simulink model "PlaneSimulationModel_withSensors_r17"  (R2022b)
settings: Solver=FixedStepAuto  StartTime=0.0  StopTime=20  FixedStep=0.0025  RelTol=1e-3
libraries: simulink x12
(part 1 of 2)
settings Model: DataDictionary=plane_sm_dictionary.sldd  EnableAccessToBaseWorkspace=off  PauseTimes=0  Creator=Marcin  LastModifiedBy=Wojtek
settings SolverCC: AlgebraicLoopSolver=TrustRegion
settings DataIOCC: ReturnWorkspaceOutputs=off
settings OptimizationCC: DefaultParameterBehavior=Inlined  UseDivisionForNetSlopeComputation=on  DefaultUnderspecifiedDataType=single  PassReuseOutputArgsAs=Individual arguments  EfficientTunableParamExpr=on
settings DebuggingCC: ParameterPrecisionLossMsg=none  ParameterTunabilityLossMsg=error  UnconnectedInputMsg=warning  UnconnectedOutputMsg=warning  UnconnectedLineMsg=warning  SFMachineParentedDataDiag=warning  ArithmeticOperatorsInVariantConditions=warning
settings HardwareCC: ProdBitPerPointer=32  ProdBitPerSizeT=32  ProdBitPerPtrDiffT=32  ProdLargestAtomicInteger=Long  ProdLargestAtomicFloat=Double  ProdWordSize=32  ProdHWDeviceType=ARM Compatible->ARM Cortex-M
settings ModelReferenceCC: EnableRefExpFcnMdlSchedulingChecks=on
settings SFSimCC: SimUseLocalCustomCode=off  MATLABDynamicMemAlloc=off  CustomCodeUndefinedFunction=UseInterfaceOnly
settings RTWCC: Description=Embedded Coder  SystemTargetFile=ert.tlc  TemplateMakefile=ert_default_tmf  GenerateReport=on  RTWUseLocalCustomCode=off  Toolchain=MinGW64 | gmake (64-bit Windows)  IncludeHyperlinkInReport=on  LaunchReport=on  GenerateTraceInfo=on  GenerateTraceReport=on  GenerateTraceReportSl=on  GenerateTraceReportSf=on  GenerateTraceReportEml=on
settings CodeAppCC: ForceParamTrailComments=on  OperatorAnnotations=on  SimulinkDataObjDesc=on  SFDataObjDesc=on  InsertBlockDesc=on
settings ERTTargetCC: TargetLangStandard=C99 (ISO)  CodeReplacementLibrary=GNU C99 extensions  SupportVariableSizeSignals=on  InlinedParameterPlacement=NonHierarchical  ERTCustomFileTemplate=example_file_process.tlc  MemSecPackage=Simulink

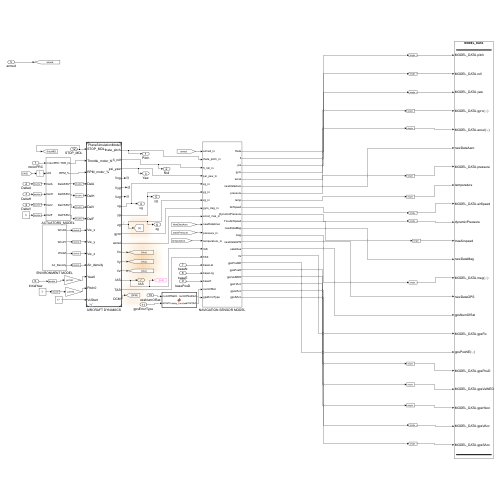
[thumbnail: Simulink's stored preview of the top-level diagram]
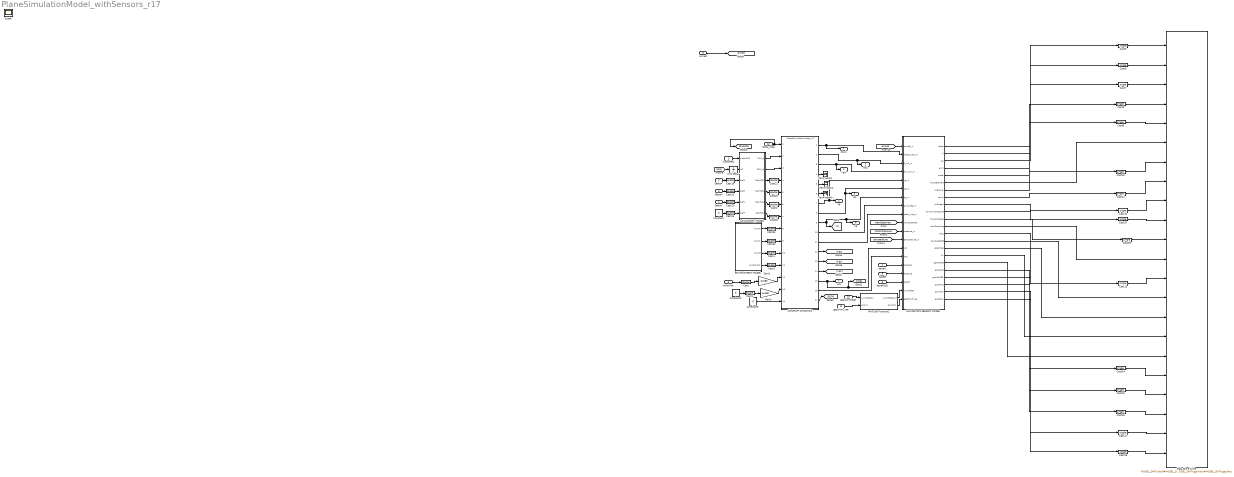
== system PlaneSimulationModel_withSensors_r17 ==
  motorPRC : Inport
  DeltaA : Inport  Port=2
  DeltaH : Inport  Port=3
  DeltaV : Inport  Port=4
  armed : Inport  Port=5  OutDataTypeStr=boolean
  InitialYaw : Inport  Port=6
  baseN : Inport  Port=7
  baseE : Inport  Port=8
  basePosD : Inport  Port=9
  gpsNumOfSat : Inport  Port=10  OutDataTypeStr=uint8
  gpsErrorType : Inport  Port=11  OutDataTypeStr=uint8
  STOP_MDL : Inport  Port=12
  ACTUATORS_MODEL : Subsystem
  AIRCRAFT DYNAMICS : ModelReference  Priority=10  ModelNameDialog=PlaneSimulationModel_r17.slx  SimulationMode=Normal  ModelReferenceVersion=11.9
  Cast{,1..4,19..24,30..32} (14 alike) : DataTypeConversion  OutDataTypeStr=double  SaturateOnIntegerOverflow=off  RndMeth=Floor
  Cast{5..18,33,37} (16 alike) : DataTypeConversion  OutDataTypeStr=single  SaturateOnIntegerOverflow=off  RndMeth=Floor
  Constant : Constant  Value=0
  Constant2 : Constant  Value=3  OutDataTypeStr=single  SampleTime=-1
  Constant6 : Constant  Value=17  OutDataTypeStr=double  SampleTime=-1
  Data Store Write : DataStoreWrite  DataStoreName=MODEL_DATA  DataStoreElements=MODEL_DATA.pitch#MODEL_DATA.roll#MODEL_DATA.yaw#MODEL_DATA.gyro(:,:)#MODEL_DATA.accel(:,:)#MODEL_DATA.newDateAero#MODEL_DATA.pressure#MODEL_DATA.temperature#MODEL_DATA.airSpeed#MODEL_DATA.dynamicPressure#MODEL_DATA.trueAirspeed#MODEL_DATA.newDataMag#MODEL_DATA.mag(:,:)#MODEL_DATA.newDataGPS#MODEL_DATA.gpsNumOfSat#MODEL_DATA.gpsFix#MODEL_DATA.gpsPosNE(:,:)#MODEL_DATA.gpsPosD#MODEL_DATA.gpsVelNED#MODEL_DATA.gpsHAcc#MODEL_DATA.gpsVAcc#MODEL_DATA.gpsSAcc  IndexOptions=Index vector (dialog)  Indices=1  OutputSizes=1
  ENVIRONMENT MODEL : Subsystem
  Gain2 : Gain  Gain=pi/180
  Gain3 : Gain  Gain=pi/180
  MATLAB Function2 : MATLAB Function  TreatAsAtomicUnit=on
  NAVIGATION SENSOR MODEL : Subsystem  Priority=50
  Terminator1 : Terminator
  Terminator2 : Terminator
  Terminator3 : Terminator
  Unit Delay : UnitDelay  SampleTime=-1  HasFrameUpgradeWarning=on
  Pitch : Outport
  Roll : Outport  Port=2
  Yaw : Outport  Port=3
  xg : Outport  Port=4
  yg : Outport  Port=5
  zg : Outport  Port=6
  IAS : Outport  Port=7
  Scope : Scope
  tag scope: StopMDL=global, armed=global
  wires:
  AIRCRAFT DYNAMICS/14 -> [Vez]
  Cast12/1 -> Data Store Write/9
  AIRCRAFT DYNAMICS/16 -> NAVIGATION SENSOR MODEL/14(TAS)
  MATLAB Function2/2(errorOut) -> NAVIGATION SENSOR MODEL/19(gpsErrorType)
  NAVIGATION SENSOR MODEL/2(fi) -> Cast6/1
  NAVIGATION SENSOR MODEL/5(accel) -> Cast9/1
  MATLAB Function2/1(numOfSatOut) -> NAVIGATION SENSOR MODEL/18(numOfSat)
  STOP_MDL/1 -> [StopMDL], AIRCRAFT DYNAMICS/1
  Cast18/1 -> Data Store Write/22
  Cast11/1 -> Data Store Write/8
  AIRCRAFT DYNAMICS/15 -> IAS/1, NAVIGATION SENSOR MODEL/13(IAS), [IAS]
  Cast33/1 -> Data Store Write/11
  baseE/1 -> NAVIGATION SENSOR MODEL/16(baseLng)
  NAVIGATION SENSOR MODEL/17(gpsPosNE) -> Data Store Write/17
  Constant6/1 -> AIRCRAFT DYNAMICS/14
  NAVIGATION SENSOR MODEL/18(gpsPosD) -> Cast14/1
  AIRCRAFT DYNAMICS/17 -> [DCM]
  NAVIGATION SENSOR MODEL/13(mag) -> Cast13/1
  AIRCRAFT DYNAMICS/12 -> [Vex]
  Cast20/1 -> AIRCRAFT DYNAMICS/5
  Cast10/1 -> Data Store Write/7
  [IAS] -> Unit Delay/1
  AIRCRAFT DYNAMICS/1 -> NAVIGATION SENSOR MODEL/2(theta_pitch_in), Pitch/1
  AIRCRAFT DYNAMICS/2 -> Roll/1, NAVIGATION SENSOR MODEL/3(fi_roll_in)
  Cast/1 -> Gain2/1
  AIRCRAFT DYNAMICS/3 -> NAVIGATION SENSOR MODEL/4(psi_yaw_in), Yaw/1
  [armed] -> NAVIGATION SENSOR MODEL/1(armed_in)
  AIRCRAFT DYNAMICS/7 -> NAVIGATION SENSOR MODEL/5(xg_in), xg/1
  [staticPressure] -> NAVIGATION SENSOR MODEL/11(pressure_in)
  AIRCRAFT DYNAMICS/11 -> NAVIGATION SENSOR MODEL/9(accel_mss_in)
  AIRCRAFT DYNAMICS/10 -> NAVIGATION SENSOR MODEL/8(gyro_deg_in)
  AIRCRAFT DYNAMICS/9 -> [z], NAVIGATION SENSOR MODEL/7(zg_in), zg/1
  NAVIGATION SENSOR MODEL/21(gpsVAcc) -> Cast17/1
  AIRCRAFT DYNAMICS/8 -> NAVIGATION SENSOR MODEL/6(yg_in), yg/1
  NAVIGATION SENSOR MODEL/4(gyro) -> Cast8/1
  gpsNumOfSat/1 -> MATLAB Function2/1(numOfSatIn)
  Cast16/1 -> Data Store Write/20
  Cast15/1 -> Data Store Write/19
  Cast13/1 -> Data Store Write/13
  Gain3/1 -> AIRCRAFT DYNAMICS/13
  Cast9/1 -> Data Store Write/5
  Cast8/1 -> Data Store Write/4
  Cast7/1 -> Data Store Write/3
  NAVIGATION SENSOR MODEL/11(TrueAirSpeed) -> Cast33/1
  NAVIGATION SENSOR MODEL/10(DynamicPressure) -> Cast37/1
  InitialYaw/1 -> Cast/1
  Cast5/1 -> Data Store Write/1
  NAVIGATION SENSOR MODEL/15(satellites) -> Data Store Write/15
  NAVIGATION SENSOR MODEL/20(gpsHAcc) -> Cast16/1
  NAVIGATION SENSOR MODEL/19(gpsVelNED) -> Cast15/1
  Cast1/1 -> Gain3/1
  NAVIGATION SENSOR MODEL/9(AirSpeed) -> Cast12/1
  NAVIGATION SENSOR MODEL/8(temp) -> Cast11/1
  NAVIGATION SENSOR MODEL/3(psi) -> Cast7/1
  NAVIGATION SENSOR MODEL/16(fix) -> Data Store Write/16
  [NewDataAreo] -> NAVIGATION SENSOR MODEL/10(newDataAreo)
  NAVIGATION SENSOR MODEL/7(pressure) -> Cast10/1
  NAVIGATION SENSOR MODEL/1(theta) -> Cast5/1
  NAVIGATION SENSOR MODEL/6(newDataAero) -> Data Store Write/6
  [temperature] -> NAVIGATION SENSOR MODEL/12(temperature_in)
  basePosD/1 -> NAVIGATION SENSOR MODEL/17(baseH)
  Cast14/1 -> Data Store Write/18
  Cast21/1 -> AIRCRAFT DYNAMICS/4
  Cast37/1 -> Data Store Write/10
  NAVIGATION SENSOR MODEL/12(newDataMag) -> Data Store Write/12
  NAVIGATION SENSOR MODEL/14(newDataGPS) -> Data Store Write/14
  gpsErrorType/1 -> MATLAB Function2/2(errorIn)
  Cast6/1 -> Data Store Write/2
  Constant2/1 -> Cast1/1
  AIRCRAFT DYNAMICS/13 -> [Vey]
  Cast17/1 -> Data Store Write/21
  baseN/1 -> NAVIGATION SENSOR MODEL/15(baseLat)
  NAVIGATION SENSOR MODEL/22(gpsSAcc) -> Cast18/1
  armed/1 -> [armed]
  AIRCRAFT DYNAMICS/4 -> Terminator1/1
  AIRCRAFT DYNAMICS/5 -> Terminator2/1
  AIRCRAFT DYNAMICS/6 -> Terminator3/1
  Cast2/1 -> AIRCRAFT DYNAMICS/6
  Gain2/1 -> AIRCRAFT DYNAMICS/12
  Cast4/1 -> AIRCRAFT DYNAMICS/10
  Cast32/1 -> AIRCRAFT DYNAMICS/9
  Cast31/1 -> AIRCRAFT DYNAMICS/8
  Cast30/1 -> AIRCRAFT DYNAMICS/7
  Cast3/1 -> AIRCRAFT DYNAMICS/11
  ENVIRONMENT MODEL/4(Air_Density) -> Cast3/1
  ENVIRONMENT MODEL/3(WindZ) -> Cast4/1
  ENVIRONMENT MODEL/2(WindY) -> Cast32/1
  ENVIRONMENT MODEL/1(WindX) -> Cast31/1
  motorPRC/1 -> ACTUATORS_MODEL/1(motorPRC)
  Unit Delay/1 -> ACTUATORS_MODEL/2(IAS)
  ACTUATORS_MODEL/1(THR_N) -> AIRCRAFT DYNAMICS/2
  ACTUATORS_MODEL/2(RPM_%) -> AIRCRAFT DYNAMICS/3
  ACTUATORS_MODEL/3(DelASRV) -> Cast21/1
  ACTUATORS_MODEL/4(DelHSRV) -> Cast20/1
  ACTUATORS_MODEL/5(DelVSRV) -> Cast2/1
  ACTUATORS_MODEL/6(DelFSRV) -> Cast30/1
  DeltaA/1 -> Cast19/1
  DeltaH/1 -> Cast22/1
  DeltaV/1 -> Cast23/1
  Constant/1 -> Cast24/1
  Cast19/1 -> ACTUATORS_MODEL/3(DelA)
  Cast22/1 -> ACTUATORS_MODEL/4(DelH)
  Cast23/1 -> ACTUATORS_MODEL/5(DelV)
  Cast24/1 -> ACTUATORS_MODEL/6(DelF)

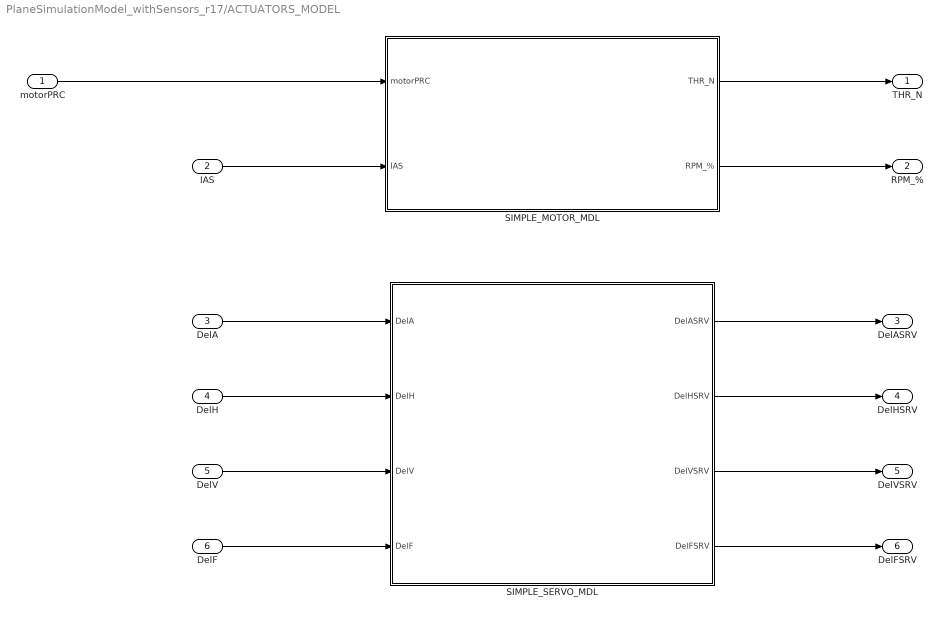
== system PlaneSimulationModel_withSensors_r17/ACTUATORS_MODEL ==
  motorPRC : Inport
  IAS : Inport  Port=2
  DelA : Inport  Port=3
  DelH : Inport  Port=4
  DelV : Inport  Port=5
  DelF : Inport  Port=6
  SIMPLE_MOTOR_MDL : Subsystem
  SIMPLE_SERVO_MDL : Subsystem
  THR_N : Outport
  RPM_% : Outport  Port=2
  DelASRV : Outport  Port=3
  DelHSRV : Outport  Port=4
  DelVSRV : Outport  Port=5
  DelFSRV : Outport  Port=6
  wires:
  SIMPLE_MOTOR_MDL/1(THR_N) -> THR_N/1
  SIMPLE_MOTOR_MDL/2(RPM_%) -> RPM_%/1
  IAS/1 -> SIMPLE_MOTOR_MDL/2(IAS)
  motorPRC/1 -> SIMPLE_MOTOR_MDL/1(motorPRC)
  DelA/1 -> SIMPLE_SERVO_MDL/1(DelA)
  SIMPLE_SERVO_MDL/1(DelASRV) -> DelASRV/1
  DelH/1 -> SIMPLE_SERVO_MDL/2(DelH)
  DelV/1 -> SIMPLE_SERVO_MDL/3(DelV)
  DelF/1 -> SIMPLE_SERVO_MDL/4(DelF)
  SIMPLE_SERVO_MDL/2(DelHSRV) -> DelHSRV/1
  SIMPLE_SERVO_MDL/3(DelVSRV) -> DelVSRV/1
  SIMPLE_SERVO_MDL/4(DelFSRV) -> DelFSRV/1

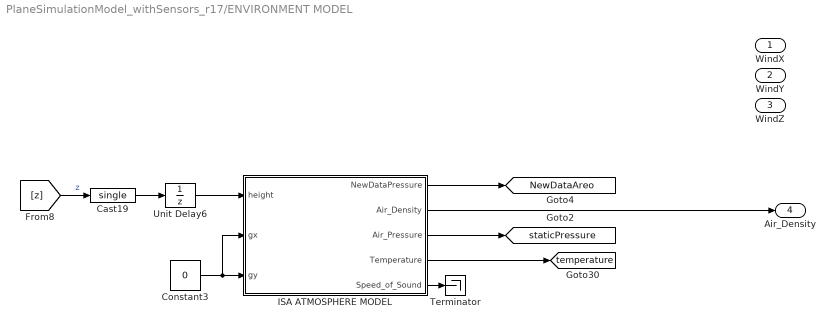
== system PlaneSimulationModel_withSensors_r17/ENVIRONMENT MODEL ==
  Cast19 : DataTypeConversion  OutDataTypeStr=single  SaturateOnIntegerOverflow=off  RndMeth=Floor
  Constant3 : Constant  Value=0  OutDataTypeStr=single  SampleTime=-1
  ISA ATMOSPHERE MODEL : MATLAB Function  TreatAsAtomicUnit=on  mask{acc_to_gravity=9.80665, ratio_heats=1.4, gas_const=287.0531, lapse_rate=0.0065, height_of_troposphere=110000, height_of_tropopause=20000, air_density=1.225, pressure_sea_level=101325, temperature_sea_level=288.15, lowest_altitude=0, frequency=100, delay=50, pressure_deviation=6, en_acc_pressure_noise=on, max_bias_value=0, max_bias_time=50, dt=0.0025}
      mask prompts: acc_to_gravity "Acceleration due to gravity (m/s^2)"; ratio_heats "Ratio of specific heats"; gas_const "Characteristic gas constant (J/Kg/K)"; lapse_rate "Lapse rate (K/m)"; height_of_troposphere "Height of troposphere (m)"; height_of_tropopause "Height of tropopause (m)"; air_density "Air density at mean sea level (Kg/m^3)"; pressure_sea_level "Ambient pressure at mean sea level (N/m^2)"; temperature_sea_level "Ambient temperature at mean sea level"; lowest_altitude "Lowest altitude (m)"; frequency "Frequency [Hz]"; delay "Latency [ms]"; pressure_deviation "Pressure Deviation [Pa]"; en_acc_pressure_noise "Enable acc pressure noise"; max_bias_value "Max pressure bias value [Pa]"; max_bias_time "Max value bias time [s]"; dt "Sample Time [s]"
  Terminator : Terminator
  Unit Delay6 : UnitDelay  SampleTime=-1  HasFrameUpgradeWarning=on
  WindX : Outport
  WindY : Outport  Port=2
  WindZ : Outport  Port=3
  Air_Density : Outport  Port=4
  tag scope: NewDataAreo=global, staticPressure=global, temperature=global
  wires:
  [z] -> Cast19/1  "z"
  ISA ATMOSPHERE MODEL/3(Air_Pressure) -> [staticPressure]
  Constant3/1 -> ISA ATMOSPHERE MODEL/2(gx), ISA ATMOSPHERE MODEL/3(gy)
  Unit Delay6/1 -> ISA ATMOSPHERE MODEL/1(height)
  ISA ATMOSPHERE MODEL/5(Speed_of_Sound) -> Terminator/1
  ISA ATMOSPHERE MODEL/1(NewDataPressure) -> [NewDataAreo]
  Cast19/1 -> Unit Delay6/1
  ISA ATMOSPHERE MODEL/4(Temperature) -> [temperature]
  ISA ATMOSPHERE MODEL/2(Air_Density) -> Air_Density/1

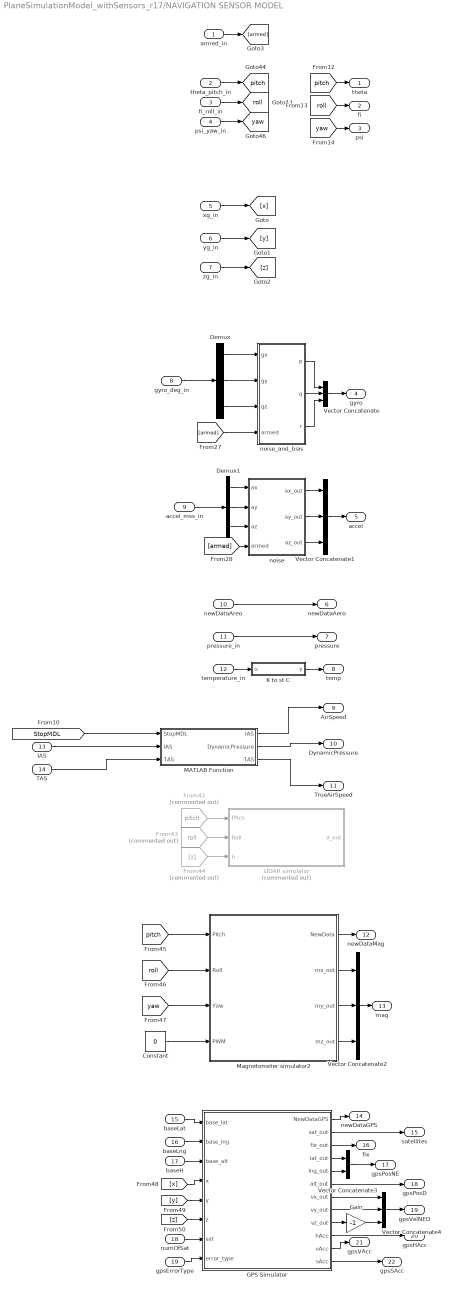
== system PlaneSimulationModel_withSensors_r17/NAVIGATION SENSOR MODEL ==
  armed_in : Inport
  theta_pitch_in : Inport  Port=2
  fi_roll_in : Inport  Port=3
  psi_yaw_in : Inport  Port=4
  xg_in : Inport  Port=5
  yg_in : Inport  Port=6
  zg_in : Inport  Port=7
  gyro_deg_in : Inport  Port=8
  accel_mss_in : Inport  Port=9
  newDataAreo : Inport  Port=10
  pressure_in : Inport  Port=11
  temperature_in : Inport  Port=12
  IAS : Inport  Port=13
  TAS : Inport  Port=14
  baseLat : Inport  Port=15
  baseLng : Inport  Port=16
  baseH : Inport  Port=17
  numOfSat : Inport  Port=18
  gpsErrorType : Inport  Port=19
  Constant : Constant  Value=0  OutDataTypeStr=double  SampleTime=-1
  Demux : Demux  Outputs=3
  Demux1 : Demux  Outputs=3
  From42 : From  Commented=on  GotoTag=pitch  TagVisibility=global
  From43 : From  Commented=on  GotoTag=roll  TagVisibility=global
  From44 : From  Commented=on  GotoTag=z  TagVisibility=global
  GPS Simulator : MATLAB Function  TreatAsAtomicUnit=on  mask{f_gps=5, gps_delay=250, sigma=1, sigma_alt=1, dt=0.0025}
      mask prompts: f_gps "GPS frequency [Hz]"; gps_delay "GPS latency [ms]"; sigma "Horizontal Standard Deviation [m]"; sigma_alt "Vertical Standard Deviation [m]"; dt "Sample Time [s]"
  Gain : Gain  Gain=-1
  K to st C : MATLAB Function  TreatAsAtomicUnit=on
  LIDAR simulator : MATLAB Function  Commented=on  TreatAsAtomicUnit=on  mask{f_lid=100, lid_delay=50, sigma=0.3, range=40, dt=0.0025}
      mask prompts: f_lid "LIDAR Frequency [Hz]"; lid_delay "LIDAR latency [ms]"; sigma "LIDAR Standard Deviation [m]"; range "LIDAR Range [m]"; dt "Sample Time [s]"
  MATLAB Function : MATLAB Function  TreatAsAtomicUnit=on
  Magnetometer simulator2 : MATLAB Function  TreatAsAtomicUnit=on  mask{f_mag=100, mag_delay=50, sigma=15, PWM_dev_min=65, PWM_bias=40, dt=0.0025}
      mask prompts: f_mag "MAG Frequency [Hz]"; mag_delay "MAG latency [ms]"; sigma "Output Standard Deviation"; PWM_dev_min "PWM_min deviation [%]"; PWM_bias "PWM bias max"; dt "Sample Time [s]"
  Vector Concatenate{,1..2,4} (4 alike) : Concatenate  NumInputs=3
  Vector Concatenate3 : Concatenate
  noise : Subsystem
  noise_and_bias : Subsystem  TreatAsAtomicUnit=on
  theta : Outport  VectorParamsAs1DForOutWhenUnconnected=off
  fi : Outport  Port=2  VectorParamsAs1DForOutWhenUnconnected=off
  psi : Outport  Port=3  VectorParamsAs1DForOutWhenUnconnected=off
  gyro : Outport  Port=4  VectorParamsAs1DForOutWhenUnconnected=off
  accel : Outport  Port=5  VectorParamsAs1DForOutWhenUnconnected=off
  newDataAero : Outport  Port=6  VectorParamsAs1DForOutWhenUnconnected=off
  pressure : Outport  Port=7  VectorParamsAs1DForOutWhenUnconnected=off
  temp : Outport  Port=8  VectorParamsAs1DForOutWhenUnconnected=off
  AirSpeed : Outport  Port=9  VectorParamsAs1DForOutWhenUnconnected=off
  DynamicPressure : Outport  Port=10  VectorParamsAs1DForOutWhenUnconnected=off
  TrueAirSpeed : Outport  Port=11  VectorParamsAs1DForOutWhenUnconnected=off
  newDataMag : Outport  Port=12  VectorParamsAs1DForOutWhenUnconnected=off
  mag : Outport  Port=13  VectorParamsAs1DForOutWhenUnconnected=off
  newDataGPS : Outport  Port=14  VectorParamsAs1DForOutWhenUnconnected=off
  satellites : Outport  Port=15  VectorParamsAs1DForOutWhenUnconnected=off
  fix : Outport  Port=16  VectorParamsAs1DForOutWhenUnconnected=off
  gpsPosNE : Outport  Port=17  VectorParamsAs1DForOutWhenUnconnected=off
  gpsPosD : Outport  Port=18  VectorParamsAs1DForOutWhenUnconnected=off
  gpsVelNED : Outport  Port=19  VectorParamsAs1DForOutWhenUnconnected=off
  gpsHAcc : Outport  Port=20  VectorParamsAs1DForOutWhenUnconnected=off
  gpsVAcc : Outport  Port=21  VectorParamsAs1DForOutWhenUnconnected=off
  gpsSAcc : Outport  Port=22  VectorParamsAs1DForOutWhenUnconnected=off
  tag scope: pitch=global, roll=global, yaw=global
  wires:
  Demux/1 -> noise_and_bias/1(gx)
  Demux/3 -> noise_and_bias/3(gz)
  [roll] -> Magnetometer simulator2/2(Roll)
  pressure_in/1 -> pressure/1
  Demux/2 -> noise_and_bias/2(gy)
  [armed] -> noise/4(armed)
  Demux1/3 -> noise/3(az)
  accel_mss_in/1 -> Demux1/1
  Demux1/2 -> noise/2(ay)
  Demux1/1 -> noise/1(ax)
  From44/1 -> LIDAR simulator/3(h)
  From42/1 -> LIDAR simulator/1(Pitch)
  From43/1 -> LIDAR simulator/2(Roll)
  Constant/1 -> Magnetometer simulator2/4(PWM)
  temperature_in/1 -> K to st C/1(u)
  K to st C/1(y) -> temp/1
  [yaw] -> Magnetometer simulator2/3(Yaw)
  [pitch] -> Magnetometer simulator2/1(Pitch)
  [armed] -> noise_and_bias/4(armed)
  fi_roll_in/1 -> [roll]
  theta_pitch_in/1 -> [pitch]
  psi_yaw_in/1 -> [yaw]
  [pitch] -> theta/1
  [roll] -> fi/1
  [yaw] -> psi/1
  gyro_deg_in/1 -> Demux/1
  xg_in/1 -> [x]
  yg_in/1 -> [y]
  zg_in/1 -> [z]
  armed_in/1 -> [armed]
  IAS/1 -> MATLAB Function/2("IAS ")
  noise_and_bias/2(q) -> Vector Concatenate/2
  noise_and_bias/1(p) -> Vector Concatenate/1
  noise_and_bias/3(r) -> Vector Concatenate/3
  Vector Concatenate/1 -> gyro/1
  noise/2(ay_out) -> Vector Concatenate1/2
  noise/1(ax_out) -> Vector Concatenate1/1
  noise/3(az_out) -> Vector Concatenate1/3
  Vector Concatenate1/1 -> accel/1
  newDataAreo/1 -> newDataAero/1
  Magnetometer simulator2/3(my_out) -> Vector Concatenate2/2
  Magnetometer simulator2/4(mz_out) -> Vector Concatenate2/3
  Vector Concatenate2/1 -> mag/1
  Magnetometer simulator2/2(mx_out) -> Vector Concatenate2/1
  Magnetometer simulator2/1(NewData) -> newDataMag/1
  GPS Simulator/12(sAcc) -> gpsSAcc/1
  Vector Concatenate3/1 -> gpsPosNE/1
  Gain/1 -> Vector Concatenate4/3
  GPS Simulator/3(fix_out) -> fix/1
  GPS Simulator/8(vy_out) -> Vector Concatenate4/2
  GPS Simulator/4(lat_out) -> Vector Concatenate3/1
  GPS Simulator/7(vx_out) -> Vector Concatenate4/1
  GPS Simulator/2(sat_out) -> satellites/1
  GPS Simulator/1(NewDataGPS) -> newDataGPS/1
  GPS Simulator/11(vAcc) -> gpsVAcc/1
  GPS Simulator/6(alt_out) -> gpsPosD/1
  GPS Simulator/9(vz_out) -> Gain/1
  GPS Simulator/5(lng_out) -> Vector Concatenate3/2
  Vector Concatenate4/1 -> gpsVelNED/1
  GPS Simulator/10(hAcc) -> gpsHAcc/1
  baseLat/1 -> GPS Simulator/1(base_lat)
  baseLng/1 -> GPS Simulator/2(base_lng)
  baseH/1 -> GPS Simulator/3(base_alt)
  [x] -> GPS Simulator/4(x)
  [y] -> GPS Simulator/5(y)
  [z] -> GPS Simulator/6(z)
  numOfSat/1 -> GPS Simulator/7(sat)
  gpsErrorType/1 -> GPS Simulator/8(error_type)
  MATLAB Function/3(TAS) -> TrueAirSpeed/1
  MATLAB Function/2(DynamicPressure) -> DynamicPressure/1
  [StopMDL] -> MATLAB Function/1(StopMDL)
  MATLAB Function/1(IAS) -> AirSpeed/1
  TAS/1 -> MATLAB Function/3("TAS ")

== system PlaneSimulationModel_withSensors_r17/ACTUATORS_MODEL/SIMPLE_MOTOR_MDL ==
  motorPRC : Inport
  IAS : Inport  Port=2
  2xelectric : Subsystem  VariantControl=(default)
  THR_N : Outport
  RPM_% : Outport  Port=2
  wires:
  [armed] -> 2xelectric/1(arm)
  motorPRC/1 -> 2xelectric/2(motorPRC)
  2xelectric/1(THR_N) -> THR_N/1
  2xelectric/2(RPM_%) -> RPM_%/1
  IAS/1 -> 2xelectric/3(IAS)

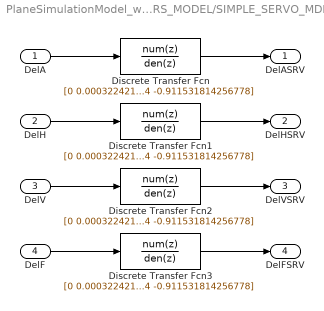
== system PlaneSimulationModel_withSensors_r17/ACTUATORS_MODEL/SIMPLE_SERVO_MDL ==
  DelA : Inport
  DelH : Inport  Port=2
  DelV : Inport  Port=3
  DelF : Inport  Port=4
  Discrete Transfer Fcn{,1..3} (4 alike) : DiscreteTransferFcn  Numerator=[0 0.000322421150918839 -0.000173176804593514]  Denominator="[1\t-1.90810999635018\t-0.0870514284817427\t1.90684266473014\t-0.911531814256778]"
  DelASRV : Outport
  DelHSRV : Outport  Port=2
  DelVSRV : Outport  Port=3
  DelFSRV : Outport  Port=4
  wires:
  DelA/1 -> Discrete Transfer Fcn/1
  DelH/1 -> Discrete Transfer Fcn1/1
  DelV/1 -> Discrete Transfer Fcn2/1
  DelF/1 -> Discrete Transfer Fcn3/1
  Discrete Transfer Fcn/1 -> DelASRV/1
  Discrete Transfer Fcn1/1 -> DelHSRV/1
  Discrete Transfer Fcn2/1 -> DelVSRV/1
  Discrete Transfer Fcn3/1 -> DelFSRV/1

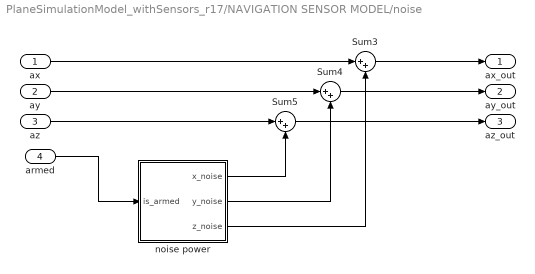
== system PlaneSimulationModel_withSensors_r17/NAVIGATION SENSOR MODEL/noise ==
  ax : Inport
  ay : Inport  Port=2
  az : Inport  Port=3
  armed : Inport  Port=4
  Sum3 : Sum  Inputs=|++
  Sum4 : Sum  Inputs=|++
  Sum5 : Sum  Inputs=|++
  noise power : Subsystem
  ax_out : Outport  VectorParamsAs1DForOutWhenUnconnected=off
  ay_out : Outport  Port=2  VectorParamsAs1DForOutWhenUnconnected=off
  az_out : Outport  Port=3  VectorParamsAs1DForOutWhenUnconnected=off
  wires:
  noise power/1(x_noise) -> Sum5/2
  Sum3/1 -> ax_out/1
  Sum4/1 -> ay_out/1
  Sum5/1 -> az_out/1
  noise power/2(y_noise) -> Sum4/2
  noise power/3(z_noise) -> Sum3/2
  az/1 -> Sum5/1
  ay/1 -> Sum4/1
  ax/1 -> Sum3/1
  armed/1 -> noise power/1(is_armed)

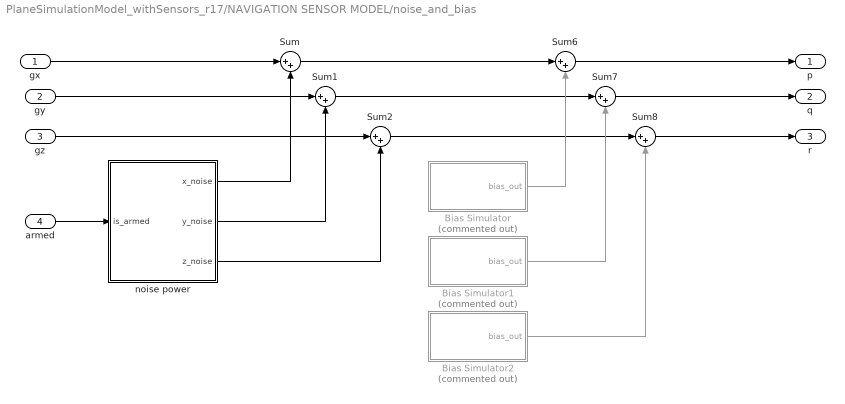
== system PlaneSimulationModel_withSensors_r17/NAVIGATION SENSOR MODEL/noise_and_bias ==
  gx : Inport
  gy : Inport  Port=2
  gz : Inport  Port=3
  armed : Inport  Port=4
  Bias Simulator : MATLAB Function  Commented=on  TreatAsAtomicUnit=on  SystemSampleTime=0.0025  mask{max_bias=0.25, max_bias_time=200, st=0.0025}
      mask prompts: max_bias "Max bias value"; max_bias_time "Max bias time [s]"; st "Sample time"
  Bias Simulator1 : MATLAB Function  Commented=on  TreatAsAtomicUnit=on  SystemSampleTime=0.0025  mask{max_bias=0.3, max_bias_time=600, st=0.0025}
      mask prompts: max_bias "Max bias value"; max_bias_time "Max bias time [s]"; st "Sample time"
  Bias Simulator2 : MATLAB Function  Commented=on  TreatAsAtomicUnit=on  SystemSampleTime=0.0025  mask{max_bias=0.32, max_bias_time=650, st=0.0025}
      mask prompts: max_bias "Max bias value"; max_bias_time "Max bias time [s]"; st "Sample time"
  Sum{,1..2,6..8} (6 alike) : Sum  Inputs=|++
  noise power : Subsystem  TreatAsAtomicUnit=on
  p : Outport  VectorParamsAs1DForOutWhenUnconnected=off
  q : Outport  Port=2  VectorParamsAs1DForOutWhenUnconnected=off
  r : Outport  Port=3  VectorParamsAs1DForOutWhenUnconnected=off
  wires:
  gx/1 -> Sum/1
  gy/1 -> Sum1/1
  gz/1 -> Sum2/1
  noise power/1(x_noise) -> Sum/2
  noise power/3(z_noise) -> Sum2/2
  noise power/2(y_noise) -> Sum1/2
  Sum/1 -> Sum6/1
  Sum1/1 -> Sum7/1
  Sum2/1 -> Sum8/1
  Bias Simulator/1(bias_out) -> Sum6/2
  Bias Simulator1/1(bias_out) -> Sum7/2
  Bias Simulator2/1(bias_out) -> Sum8/2
  Sum6/1 -> p/1
  Sum7/1 -> q/1
  Sum8/1 -> r/1
  armed/1 -> noise power/1(is_armed)

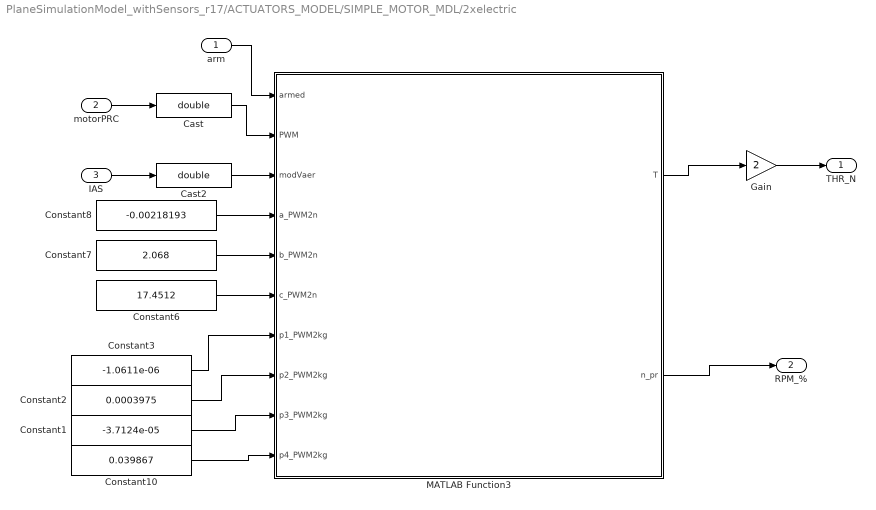
== system PlaneSimulationModel_withSensors_r17/ACTUATORS_MODEL/SIMPLE_MOTOR_MDL/2xelectric ==
  arm : Inport
  motorPRC : Inport  Port=2
  IAS : Inport  Port=3
  Cast : DataTypeConversion  OutDataTypeStr=double  SaturateOnIntegerOverflow=off  RndMeth=Floor
  Cast2 : DataTypeConversion  OutDataTypeStr=double  SaturateOnIntegerOverflow=off  RndMeth=Floor
  Constant1 : Constant  Value=-3.7124e-05  OutDataTypeStr=double  SampleTime=-1
  Constant10 : Constant  Value=0.039867  OutDataTypeStr=double  SampleTime=-1
  Constant2 : Constant  Value=0.0003975  OutDataTypeStr=double  SampleTime=-1
  Constant3 : Constant  Value=-1.0611e-06  OutDataTypeStr=double  SampleTime=-1
  Constant6 : Constant  Value=17.4512  OutDataTypeStr=double  SampleTime=-1
  Constant7 : Constant  Value=2.068  OutDataTypeStr=double  SampleTime=-1
  Constant8 : Constant  Value=-0.00218193  OutDataTypeStr=double  SampleTime=-1
  Gain : Gain  Gain=2
  MATLAB Function3 : MATLAB Function  TreatAsAtomicUnit=on
  THR_N : Outport
  RPM_% : Outport  Port=2
  wires:
  IAS/1 -> Cast2/1
  Constant7/1 -> MATLAB Function3/5(b_PWM2n)
  motorPRC/1 -> Cast/1
  Constant8/1 -> MATLAB Function3/4(a_PWM2n)
  arm/1 -> MATLAB Function3/1(armed)
  Cast/1 -> MATLAB Function3/2(PWM)
  Constant6/1 -> MATLAB Function3/6(c_PWM2n)
  MATLAB Function3/2(n_pr) -> RPM_%/1
  MATLAB Function3/1(T) -> Gain/1
  Gain/1 -> THR_N/1
  Cast2/1 -> MATLAB Function3/3(modVaer)
  Constant10/1 -> MATLAB Function3/10(p4_PWM2kg)
  Constant1/1 -> MATLAB Function3/9(p3_PWM2kg)
  Constant2/1 -> MATLAB Function3/8(p2_PWM2kg)
  Constant3/1 -> MATLAB Function3/7(p1_PWM2kg)

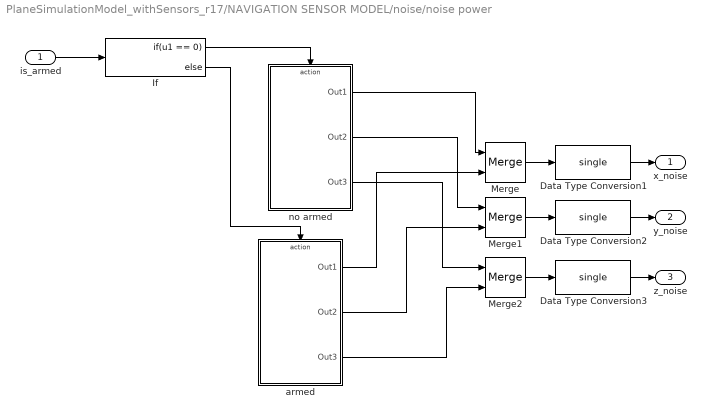
== system PlaneSimulationModel_withSensors_r17/NAVIGATION SENSOR MODEL/noise/noise power ==
  is_armed : Inport
  Data Type Conversion1 : DataTypeConversion  OutDataTypeStr=single  SaturateOnIntegerOverflow=off  RndMeth=Floor
  Data Type Conversion2 : DataTypeConversion  OutDataTypeStr=single  SaturateOnIntegerOverflow=off  RndMeth=Floor
  Data Type Conversion3 : DataTypeConversion  OutDataTypeStr=single  SaturateOnIntegerOverflow=off  RndMeth=Floor
  If : If  IfExpression=u1 == 0
  Merge : Merge
  Merge1 : Merge
  Merge2 : Merge
  armed : Subsystem  TreatAsAtomicUnit=on
  no armed : Subsystem  TreatAsAtomicUnit=on
  x_noise : Outport  VectorParamsAs1DForOutWhenUnconnected=off
  y_noise : Outport  Port=2  VectorParamsAs1DForOutWhenUnconnected=off
  z_noise : Outport  Port=3  VectorParamsAs1DForOutWhenUnconnected=off
  wires:
  Merge2/1 -> Data Type Conversion3/1
  Merge1/1 -> Data Type Conversion2/1
  Merge/1 -> Data Type Conversion1/1
  is_armed/1 -> If/1
  If/1 -> no armed/Action
  no armed/1(Out1) -> Merge/1
  no armed/2(Out2) -> Merge1/1
  no armed/3(Out3) -> Merge2/1
  If/2 -> armed/Action
  armed/1(Out1) -> Merge/2
  armed/2(Out2) -> Merge1/2
  armed/3(Out3) -> Merge2/2
  Data Type Conversion2/1 -> y_noise/1
  Data Type Conversion3/1 -> z_noise/1
  Data Type Conversion1/1 -> x_noise/1

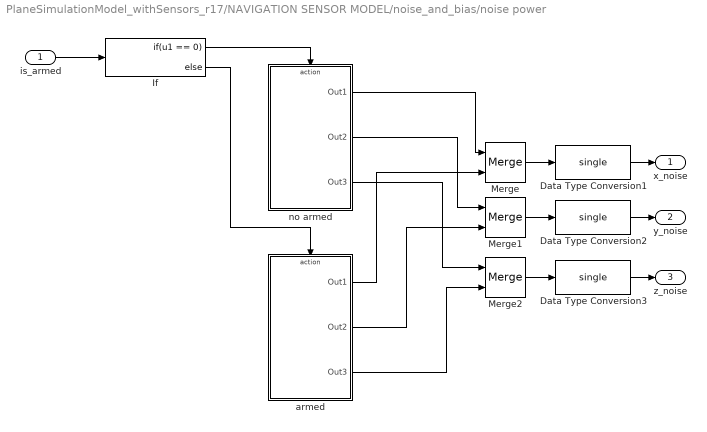
== system PlaneSimulationModel_withSensors_r17/NAVIGATION SENSOR MODEL/noise_and_bias/noise power ==
  is_armed : Inport
  Data Type Conversion1 : DataTypeConversion  OutDataTypeStr=single  SaturateOnIntegerOverflow=off  RndMeth=Floor
  Data Type Conversion2 : DataTypeConversion  OutDataTypeStr=single  SaturateOnIntegerOverflow=off  RndMeth=Floor
  Data Type Conversion3 : DataTypeConversion  OutDataTypeStr=single  SaturateOnIntegerOverflow=off  RndMeth=Floor
  If : If  IfExpression=u1 == 0
  Merge : Merge
  Merge1 : Merge
  Merge2 : Merge
  armed : Subsystem  TreatAsAtomicUnit=on
  no armed : Subsystem  TreatAsAtomicUnit=on
  x_noise : Outport  VectorParamsAs1DForOutWhenUnconnected=off
  y_noise : Outport  Port=2  VectorParamsAs1DForOutWhenUnconnected=off
  z_noise : Outport  Port=3  VectorParamsAs1DForOutWhenUnconnected=off
  wires:
  Merge2/1 -> Data Type Conversion3/1
  Merge1/1 -> Data Type Conversion2/1
  Merge/1 -> Data Type Conversion1/1
  is_armed/1 -> If/1
  If/1 -> no armed/Action
  no armed/1(Out1) -> Merge/1
  no armed/2(Out2) -> Merge1/1
  no armed/3(Out3) -> Merge2/1
  If/2 -> armed/Action
  armed/1(Out1) -> Merge/2
  armed/2(Out2) -> Merge1/2
  armed/3(Out3) -> Merge2/2
  Data Type Conversion2/1 -> y_noise/1
  Data Type Conversion3/1 -> z_noise/1
  Data Type Conversion1/1 -> x_noise/1

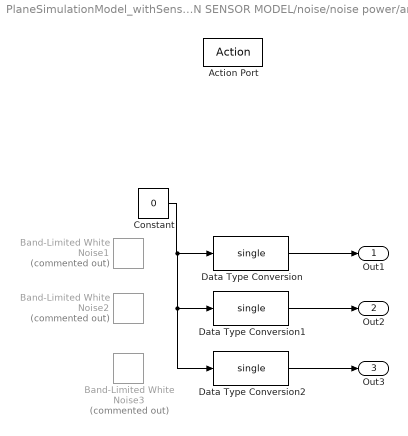
== system PlaneSimulationModel_withSensors_r17/NAVIGATION SENSOR MODEL/noise/noise power/armed ==
  Action Port : ActionPort  ActionPortLabel=else
  Band-Limited White Noise1 : simulink/Sources/Band-Limited White Noise  Commented=on  Cov=[0.0002]  Ts=0.0025  seed=[23341]
  Band-Limited White Noise2 : simulink/Sources/Band-Limited White Noise  Commented=on  Cov=[0.0002]  Ts=0.0025  seed=[20301]
  Band-Limited White Noise3 : simulink/Sources/Band-Limited White Noise  Commented=on  Cov=[0.0002]  Ts=0.0025  seed=[14368]
  Constant : Constant  Value=0  OutDataTypeStr=single  SampleTime=-1
  Data Type Conversion : DataTypeConversion  OutDataTypeStr=single  SaturateOnIntegerOverflow=off  RndMeth=Floor
  Data Type Conversion1 : DataTypeConversion  OutDataTypeStr=single  SaturateOnIntegerOverflow=off  RndMeth=Floor
  Data Type Conversion2 : DataTypeConversion  OutDataTypeStr=single  SaturateOnIntegerOverflow=off  RndMeth=Floor
  Out1 : Outport  VectorParamsAs1DForOutWhenUnconnected=off
  Out2 : Outport  Port=2  VectorParamsAs1DForOutWhenUnconnected=off
  Out3 : Outport  Port=3  VectorParamsAs1DForOutWhenUnconnected=off
  wires:
  Constant/1 -> Data Type Conversion2/1, Data Type Conversion1/1, Data Type Conversion/1
  Data Type Conversion/1 -> Out1/1
  Data Type Conversion1/1 -> Out2/1
  Data Type Conversion2/1 -> Out3/1

== system PlaneSimulationModel_withSensors_r17/NAVIGATION SENSOR MODEL/noise/noise power/no armed ==
  Action Port : ActionPort  ActionPortLabel=if(u1 == 0)
  Band-Limited White Noise1 : simulink/Sources/Band-Limited White Noise  Cov=[0.000002]  Ts=0.0025  seed=[23341]
  Band-Limited White Noise2 : simulink/Sources/Band-Limited White Noise  Cov=[0.000002]  Ts=0.0025  seed=[20301]
  Band-Limited White Noise3 : simulink/Sources/Band-Limited White Noise  Cov=[0.000002]  Ts=0.0025  seed=[14368]
  Data Type Conversion : DataTypeConversion  OutDataTypeStr=single  SaturateOnIntegerOverflow=off  RndMeth=Floor
  Data Type Conversion1 : DataTypeConversion  OutDataTypeStr=single  SaturateOnIntegerOverflow=off  RndMeth=Floor
  Data Type Conversion2 : DataTypeConversion  OutDataTypeStr=single  SaturateOnIntegerOverflow=off  RndMeth=Floor
  Out1 : Outport  VectorParamsAs1DForOutWhenUnconnected=off
  Out2 : Outport  Port=2  VectorParamsAs1DForOutWhenUnconnected=off
  Out3 : Outport  Port=3  VectorParamsAs1DForOutWhenUnconnected=off
  wires:
  Band-Limited White Noise3/1 -> Data Type Conversion2/1
  Band-Limited White Noise2/1 -> Data Type Conversion1/1
  Band-Limited White Noise1/1 -> Data Type Conversion/1
  Data Type Conversion/1 -> Out1/1
  Data Type Conversion1/1 -> Out2/1
  Data Type Conversion2/1 -> Out3/1

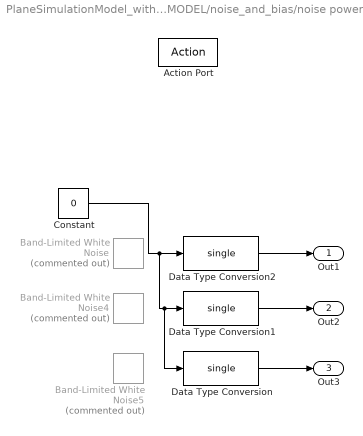
== system PlaneSimulationModel_withSensors_r17/NAVIGATION SENSOR MODEL/noise_and_bias/noise power/armed ==
  Action Port : ActionPort  ActionPortLabel=else
  Band-Limited White Noise : simulink/Sources/Band-Limited White Noise  Commented=on  Cov=[0.00001]  Ts=0.0025  seed=[-341]
  Band-Limited White Noise4 : simulink/Sources/Band-Limited White Noise  Commented=on  Cov=[0.00001]  Ts=0.0025  seed=[-321]
  Band-Limited White Noise5 : simulink/Sources/Band-Limited White Noise  Commented=on  Cov=[0.00001]  Ts=0.0025  seed=[-331]
  Constant : Constant  Value=0  OutDataTypeStr=single  SampleTime=-1
  Data Type Conversion : DataTypeConversion  OutDataTypeStr=single  SaturateOnIntegerOverflow=off  RndMeth=Floor
  Data Type Conversion1 : DataTypeConversion  OutDataTypeStr=single  SaturateOnIntegerOverflow=off  RndMeth=Floor
  Data Type Conversion2 : DataTypeConversion  OutDataTypeStr=single  SaturateOnIntegerOverflow=off  RndMeth=Floor
  Out1 : Outport  VectorParamsAs1DForOutWhenUnconnected=off
  Out2 : Outport  Port=2  VectorParamsAs1DForOutWhenUnconnected=off
  Out3 : Outport  Port=3  VectorParamsAs1DForOutWhenUnconnected=off
  wires:
  Constant/1 -> Data Type Conversion/1, Data Type Conversion1/1, Data Type Conversion2/1
  Data Type Conversion/1 -> Out3/1
  Data Type Conversion1/1 -> Out2/1
  Data Type Conversion2/1 -> Out1/1

== system PlaneSimulationModel_withSensors_r17/NAVIGATION SENSOR MODEL/noise_and_bias/noise power/no armed ==
  Action Port : ActionPort  ActionPortLabel=if(u1 == 0)
  Band-Limited White Noise : simulink/Sources/Band-Limited White Noise  Cov=[0.0000001]  Ts=0.0025  seed=[-341]
  Band-Limited White Noise4 : simulink/Sources/Band-Limited White Noise  Cov=[0.0000001]  Ts=0.0025  seed=[-321]
  Band-Limited White Noise5 : simulink/Sources/Band-Limited White Noise  Cov=[0.0000001]  Ts=0.0025  seed=[-331]
  Data Type Conversion : DataTypeConversion  OutDataTypeStr=single  SaturateOnIntegerOverflow=off  RndMeth=Floor
  Data Type Conversion1 : DataTypeConversion  OutDataTypeStr=single  SaturateOnIntegerOverflow=off  RndMeth=Floor
  Data Type Conversion2 : DataTypeConversion  OutDataTypeStr=single  SaturateOnIntegerOverflow=off  RndMeth=Floor
  Out1 : Outport  VectorParamsAs1DForOutWhenUnconnected=off
  Out2 : Outport  Port=2  VectorParamsAs1DForOutWhenUnconnected=off
  Out3 : Outport  Port=3  VectorParamsAs1DForOutWhenUnconnected=off
  wires:
  Band-Limited White Noise4/1 -> Data Type Conversion1/1
  Band-Limited White Noise/1 -> Data Type Conversion/1
  Band-Limited White Noise5/1 -> Data Type Conversion2/1
  Data Type Conversion/1 -> Out1/1
  Data Type Conversion1/1 -> Out2/1
  Data Type Conversion2/1 -> Out3/1

== matlab function PlaneSimulationModel_withSensors_r17/NAVIGATION SENSOR MODEL/LIDAR simulator ==
  data: Pitch input; d_out output; Roll input; h input; dt parameter single; lid_delay parameter single; f_lid parameter single; sigma parameter; range parameter
function d_out  = fcn(Pitch,Roll,h,dt, lid_delay, f_lid,sigma,range)
persistent zoh; if isempty(zoh) zoh=single(0);end
persistent init; if isempty(init) init=false;end
persistent d_delay; if isempty(d_delay) d_delay=single(0);end
persistent ile_probek_delay; if isempty(ile_probek_delay) ile_probek_delay=single(0);end
persistent ile_probek_zoh; if isempty(ile_probek_zoh) ile_probek_zoh=single(0);end
persistent i; if isempty(i) i=single(0);end
persistent x_out; if isempty(x_out) x_out=single(0);end
persistent buff; if isempty(buff) buff=single(zeros(12,3));end
% dt = single(0.004); %[s]
% gps_delay = single(200); %[ms]
% f_mag = single(5); % [Hz]
% base_lat = single(52.251045);
% base_lng = single(20.935379);

if(~init)
    init=true;
    ile_probek_zoh = 1/single(f_lid)/single(dt);
    ile_probek_delay = single(lid_delay)*0.001/(1/single(f_lid))+1;
    
end

    cp = cosd(Pitch);
    cr = cosd(Roll);

       
    %Macierz przejscia z ukladu inercjalnego (zwiazanego z ziemia) do ukladu 
    %zwiazanego z obiektem na potrzeby warunków początkowych 
    Lqg = cp*cr;
   
    if(zoh>ile_probek_zoh-1)
        i=i+1;
        if(i>ile_probek_delay)
            i=single(1);
        end

       
        r_h = sigma*rand(1,1,'single');
        h = h + r_h;
        if(h<=0)
            h=single(0);
        end
        if(Lqg>0)
            d=h/Lqg;
        else
            d=single(0);
        end
       
        if(d>range || d<=0)
            d=single(0);
        end
       
        buff(i,1)=d(1);
        
        zoh=single(0);
        if(i+1>ile_probek_delay)
            d_delay=buff(1,1);
        else
            d_delay=buff(i+1,1);
        end

   end
zoh=zoh+1;


d_out = d_delay;

== matlab function PlaneSimulationModel_withSensors_r17/NAVIGATION SENSOR MODEL/noise_and_bias/Bias Simulator ==
  data: bias_out output; max_bias parameter single size=1; st parameter single size=1; max_bias_time parameter single size=1
function bias_out = fcn(max_bias, st, max_bias_time)
%#codegen

persistent counter; if(isempty(counter)) counter = single(1); end
persistent max; if(isempty(max)) max = false; end


if(max ==false)
    counter = counter + single(0.0043/max_bias_time/0.0025 * st);
    y = reallog(single(counter));
    if(y > 1)
        y = single(1);
        max = true;
    end
else
    y = single(1);
end



bias_out = skalowanie(0,1,0,max_bias,y);

== matlab function PlaneSimulationModel_withSensors_r17/NAVIGATION SENSOR MODEL/noise_and_bias/Bias Simulator1 ==
  data: bias_out output; max_bias parameter single size=1; st parameter single size=1; max_bias_time parameter single size=1
function bias_out = fcn(max_bias, st, max_bias_time)
%#codegen

persistent counter; if(isempty(counter)) counter = single(1); end
persistent max; if(isempty(max)) max = false; end


if(max ==false)
    counter = counter + single(0.0043/max_bias_time/0.0025 * st);
    y = reallog(single(counter));
    if(y > 1)
        y = single(1);
        max = true;
    end
else
    y = single(1);
end



bias_out = skalowanie(0,1,0,max_bias,y);

== matlab function PlaneSimulationModel_withSensors_r17/NAVIGATION SENSOR MODEL/noise_and_bias/Bias Simulator2 ==
  data: bias_out output; max_bias parameter single size=1; st parameter single size=1; max_bias_time parameter single size=1
function bias_out = fcn(max_bias, st, max_bias_time)
%#codegen

persistent counter; if(isempty(counter)) counter = single(1); end
persistent max; if(isempty(max)) max = false; end


if(max ==false)
    counter = counter + single(0.0043/max_bias_time/0.0025 * st);
    y = reallog(single(counter));
    if(y > 1)
        y = single(1);
        max = true;
    end
else
    y = single(1);
end



bias_out = skalowanie(0,1,0,max_bias,y);

== matlab function PlaneSimulationModel_withSensors_r17/MATLAB Function2 ==
  data: numOfSatOut output; numOfSatIn input; errorIn input; errorOut output
function [numOfSatOut, errorOut] = delay_functon(numOfSatIn, errorIn)



persistent gpsParams;
if isempty(gpsParams)
    gpsParams = struct("numOfSat",uint8(0),...
        "error",uint8(0),...
        "crcValue", double(0), ...
        "timeAfterChange", single(0));
end

dt = single(0.0025);

crc = double(numOfSatIn) + double(errorIn);
if(crc ~= gpsParams.crcValue)
    gpsParams.crcValue = crc;
    gpsParams.timeAfterChange = single(0);
end

if(gpsParams.timeAfterChange <= 5)
    gpsParams.timeAfterChange = gpsParams.timeAfterChange + single(dt);
else
    gpsParams.numOfSat = numOfSatIn;
    gpsParams.error = errorIn;
end

numOfSatOut = gpsParams.numOfSat;
errorOut = gpsParams.error;

== matlab function PlaneSimulationModel_withSensors_r17/NAVIGATION SENSOR MODEL/MATLAB Function ==
  data: StopMDL input; IAS output; IAS input; DynamicPressure output; TAS input; TAS output
function [IAS, DynamicPressure, TAS]= IasToDynamicPressure(StopMDL, IAS, TAS)

ratio = double(2);
ro = double(1.23);

if(StopMDL == false)
    DynamicPressure = double(IAS*IAS / (ratio/ro));
else
    DynamicPressure = double(0);
    IAS = double(0);
    TAS = double(0);
end


end

== matlab function PlaneSimulationModel_withSensors_r17/ACTUATORS_MODEL/SIMPLE_MOTOR_MDL/2xelectric/MATLAB Function3 ==
  data: armed input; PWM input; modVaer input; T output; n_pr output; a_PWM2n input; b_PWM2n input; c_PWM2n input; p1_PWM2kg input; p2_PWM2kg input; p3_PWM2kg input; p4_PWM2kg input
function [T,n_pr] = fcn(armed,PWM,modVaer, a_PWM2n, b_PWM2n, c_PWM2n, p1_PWM2kg, p2_PWM2kg, p3_PWM2kg, p4_PWM2kg)

if(PWM>=10 && armed == true)
    n = a_PWM2n*PWM^2 + b_PWM2n*PWM + c_PWM2n;
    n_pr = (n/(a_PWM2n*100^2 + b_PWM2n*100 + c_PWM2n))* 100;

    T = (p1_PWM2kg*PWM^3 + p2_PWM2kg*PWM^2 + p3_PWM2kg*PWM^1 + p4_PWM2kg) * 9.81;
    T = T - modVaer*0.65;
    if(T <= 0)
        T=double(0);
    end
    
else
    T=double(0);
    n_pr = double(0);
end

== matlab function PlaneSimulationModel_withSensors_r17/NAVIGATION SENSOR MODEL/K to st C ==
  data: u input; y output
function y = fcn(u)

y = u-273.15;

== matlab function PlaneSimulationModel_withSensors_r17/ENVIRONMENT MODEL/ISA ATMOSPHERE MODEL ==
  data: NewDataPressure output; Air_Density output single; Air_Pressure output single; height input single; Temperature output single; Speed_of_Sound output single; acc_to_gravity parameter single; ratio_heats parameter single; gas_const parameter single; lapse_rate parameter single; height_of_troposphere parameter single; height_of_tropopause parameter single; air_density parameter single; pressure_sea_level parameter single; temperature_sea_level parameter single; lowest_altitude parameter single; frequency parameter single; delay parameter single; dt parameter single; en_acc_pressure_noise parameter single; gx input single; gy input single; pressure_deviation parameter single; max_bias_value parameter single; max_bias_time parameter single
function [NewDataPressure, Air_Density, Air_Pressure, Temperature, Speed_of_Sound] = Atmosphere_model(height, acc_to_gravity, ratio_heats, gas_const, lapse_rate, height_of_troposphere, height_of_tropopause, air_density, pressure_sea_level, temperature_sea_level, lowest_altitude, frequency, delay, dt, en_acc_pressure_noise, gx, gy, pressure_deviation, max_bias_value, max_bias_time)

persistent zoh; if isempty(zoh) zoh=single(0);end
persistent init; if isempty(init) init=false;end
persistent ile_probek_delay; if isempty(ile_probek_delay) ile_probek_delay=single(0);end
persistent ile_probek_zoh; if isempty(ile_probek_zoh) ile_probek_zoh=single(0);end

persistent Air_Density_dalay; if isempty(Air_Density_dalay) Air_Density_dalay=single(0);end
persistent Air_Pressure_dalay; if isempty(Air_Pressure_dalay) Air_Pressure_dalay=single(0);end
persistent Temperature_dalay; if isempty(Temperature_dalay) Temperature_dalay=single(0);end
persistent Speed_of_Sound_dalay; if isempty(Speed_of_Sound_dalay) Speed_of_Sound_dalay=single(0);end

persistent Air_Density_tmp; if isempty(Air_Density_tmp) Air_Density_tmp=single(0);end
persistent Air_Pressure_tmp; if isempty(Air_Pressure_tmp) Air_Pressure_tmp=single(0);end
persistent Temperature_tmp; if isempty(Temperature_tmp) Temperature_tmp=single(0);end
persistent Speed_of_Sound_tmp; if isempty(Speed_of_Sound_tmp) Speed_of_Sound_tmp=single(0);end

persistent i; if isempty(i) i=single(0);end
persistent buff; if isempty(buff) buff=single(zeros(12,4));end


persistent gx_lpf; if isempty(gx_lpf) gx_lpf = single(0); end
persistent gy_lpf; if isempty(gy_lpf) gy_lpf = single(0); end
    
persistent counter_bias; if(isempty(counter_bias)) counter_bias = single(1); end
persistent max_bias; if(isempty(max_bias)) max_bias = false; end 

%%
% %Acceleration due to gravity (m/s^2)
% acc_to_gravity = single(9.80665);
% 
% %Ratio of specific heats:
% ratio_heats = single(1.4);
% 
% %Characteristic gas constant (J/Kg/K)
% gas_const = single(287.0531);
% 
% %Lapse rate (K/m)
% lapse_rate = single(0.0065);
% 
% %Height of troposphere (m)
% height_of_troposphere = single(110000);
% 
% %Height of tropopause (m)
% height_of_tropopause = single(20000);
% 
% %Air density at mean sea level (Kg/m^3)
% air_density = single(1.225);
% 
% %Ambient pressure at mean sea level (N/m^2)
% pressure_sea_level = single(101325);
% 
% %Ambient temperature at mean sea level
% temperature_sea_level = single(288.15);
% 
% %Lowest altitude (m)
% lowest_altitude = single(0);

%%

if(~init)
    init=true;
    ile_probek_zoh = 1/single(1)/single(dt)/single(frequency);
    ile_probek_delay = single(delay)*0.001/(1/single(frequency))+1;
end


if (height <= 0)
    height = single(0);
end

% for en_acc_pressure_noise
gx_lpf = DigitalLPF(gx, gx_lpf, 0.2, 0.0025);
gy_lpf = DigitalLPF(gy, gy_lpf, 0.2, 0.0025);
%
pressure_deviation = pressure_deviation/2;


NewDataPressure = uint8(0);

if(zoh>ile_probek_zoh-1)
    i=i+1;
    if(i>ile_probek_delay)
        i=single(1);
    end
    NewDataPressure = uint8(1);
        
    %limit altitude to troposhere
    height_limit_troposhere = single(height);
    if (height_limit_troposhere > height_of_troposphere)
        height_limit_troposhere = height_of_troposphere;
    elseif (height_limit_troposhere < lowest_altitude)
        height_limit_troposhere = lowest_altitude;
    end

    height_limit_troposhere = height_limit_troposhere * lapse_rate;

    height_limit_troposhere = - height_limit_troposhere + temperature_sea_level;

    Temperature_tmp= height_limit_troposhere;

    temp = height_limit_troposhere*ratio_heats*gas_const;
    if(temp == 0)
        Speed_of_Sound_tmp = sqrt(temp);
    else
        Speed_of_Sound_tmp = single(0);
    end

    value_1 = height_limit_troposhere / temperature_sea_level;

    value_11 = value_1^(acc_to_gravity/(lapse_rate*gas_const));
    value_2 = value_11 * pressure_sea_level;
    value_12 = (value_11/value_1) * air_density;



    value_3 = height_of_tropopause - height;

    if(value_3 > 0)
        value_3 = single(0);
    elseif (value_3 < (height_of_troposphere - height_of_tropopause))
        value_3 = height_of_troposphere - height_of_tropopause;
    end


    value_3 = value_3 * acc_to_gravity / gas_const;

    value_3 = exp(value_3/ Temperature_tmp);


    Air_Pressure_tmp = value_2 * value_3;

    Air_Density_tmp = value_3 * value_12;
    
    %acc_pressure_noise
    if(en_acc_pressure_noise)
        acc_pressure_noise = abs(ograniczenie(gx_lpf/2, -30, 30)) + abs(ograniczenie(gy_lpf/2, -30, 30));
    else
        acc_pressure_noise = single(0);
    end
    
    % noise pressure
    rand_pressere = -pressure_deviation + (pressure_deviation+pressure_deviation)*rand(1,1, 'single');
    
    
    %bias pressure
    if(max_bias ==false)
        counter_bias = counter_bias + single(0.0043/max_bias_time/0.0025 * 1/frequency);
        bias = reallog(single(counter_bias));
        if(bias > 1)
            bias = single(1);
            max_bias = true;
        end
    else
        bias = single(1);
    end
    bias_pressure = skalowanie(0,1,0,max_bias_value,bias,0);

    
    buff(i,1)= Air_Density_tmp;
    buff(i,2)= Air_Pressure_tmp + rand_pressere + acc_pressure_noise + bias_pressure;
    buff(i,3)= Temperature_tmp;
    buff(i,4)= Speed_of_Sound_tmp;
    
    zoh=single(0);
    if(i+1>ile_probek_delay)
        Air_Density_dalay = buff(1,1);
        Air_Pressure_dalay = buff(1,2);
        Temperature_dalay = buff(1,3);
        Speed_of_Sound_dalay = buff(1,4);
    else
        Air_Density_dalay = buff(i+1,1);
        Air_Pressure_dalay = buff(i+1,2);
        Temperature_dalay = buff(i+1,3);
        Speed_of_Sound_dalay = buff(i+1,4);
    end
end
zoh=zoh+1;



Air_Density = Air_Density_dalay;
Air_Pressure = Air_Pressure_dalay;
Temperature = Temperature_dalay;
Speed_of_Sound = Speed_of_Sound_dalay;

== matlab function PlaneSimulationModel_withSensors_r17/NAVIGATION SENSOR MODEL/Magnetometer simulator2 ==
  data: NewData output; Pitch input; mx_out output; Roll input; Yaw input; my_out output; dt parameter double; mag_delay parameter double; f_mag parameter double; sigma parameter; mz_out output; PWM input double size=1; PWM_dev_min parameter double size=1; PWM_bias parameter double size=1
function [NewData, mx_out,my_out,mz_out] = fcn(Pitch,Roll,Yaw, dt, mag_delay, f_mag,sigma, PWM, PWM_dev_min, PWM_bias)
persistent zoh; if isempty(zoh) zoh=double(0);end
persistent init; if isempty(init) init=false;end
persistent mx; if isempty(mx) mx=double(0);end
persistent my; if isempty(my) my=double(0);end
persistent mz; if isempty(mz) mz=double(0);end
persistent ile_probek_delay; if isempty(ile_probek_delay) ile_probek_delay=double(0);end
persistent ile_probek_zoh; if isempty(ile_probek_zoh) ile_probek_zoh=double(0);end
persistent i; if isempty(i) i=double(0);end
persistent x_out; if isempty(x_out) x_out=double(0);end
persistent buff; if isempty(buff) buff=double(zeros(12,3));end
% dt = double(0.004); %[s]
% gps_delay = double(200); %[ms]
% f_mag = double(5); % [Hz]
% base_lat = double(52.251045);
% base_lng = double(20.935379);



sigma = sigma/2;

if(~init)
    init=true;
    ile_probek_zoh = 1/double(f_mag)/double(dt);
    ile_probek_delay = double(mag_delay)*0.001/(1/double(f_mag))+1;
    
end

NewData = uint8(0);

sp = sind(Pitch);
sr = sind(Roll);
sy = sind(0);
cp = cosd(Pitch);
cr = cosd(Roll);
cy = cosd(0);

%Macierz przejscia z ukladu inercjalnego (zwiazanego z ziemia) do ukladu 
%zwiazanego z obiektem na potrzeby warunków początkowych 
Lqg = [cy*cp              sy*cp               -sp;...
       cy*sp*sr-sy*cr     sy*sp*sr+cy*cr      cp*sr;...
       cy*sp*cr+sy*sr     sy*sp*cr-cy*sr      cp*cr];

   
if(zoh>ile_probek_zoh-1)
    i=i+1;
    if(i>ile_probek_delay)
        i=double(1);
    end

    NewData = uint8(1);
    tmp=tand(Yaw);

    if(Yaw<-90 && Yaw>-180)
        myg=-sqrt(tmp^2/(1+tmp^2));
        mxg=-sqrt(1-myg^2);
    elseif(Yaw>-90 && Yaw<=0)
        myg=-sqrt(tmp^2/(1+tmp^2));
        mxg=sqrt(1-myg^2);
    elseif(Yaw<90 && Yaw>0)
        myg=sqrt(tmp^2/(1+tmp^2));
        mxg=sqrt(1-myg^2);
    elseif(Yaw>90 && Yaw<180)
        myg=sqrt(tmp^2/(1+tmp^2));
        mxg=-sqrt(1-myg^2);
    elseif(Yaw==180 || Yaw==-180)
        myg=double(0);
        mxg=double(-1);
    elseif(Yaw==90)
        myg=double(1);
        mxg=double(0);
    elseif(Yaw==-90)
        myg=double(-1);
        mxg=double(0);
    else
        myg=double(0);
        mxg=double(0);
    end
    mzg=0;

    mod=sqrt(mxg^2+myg^2);

    myg=myg/mod*500;
    mxg=mxg/mod*500;

    tmp=Lqg*[mxg;myg;mzg];
    rand1 = -sigma + (sigma+sigma)*rand(1,1,'double');
    rand2 = -sigma + (sigma+sigma)*rand(1,1,'double');
    rand3 = -sigma + (sigma+sigma)*rand(1,1,'double');

    if((PWM - PWM_dev_min/100)> 0)
        PWM = (PWM - PWM_dev_min/100);
    else
        PWM = double(0);
    end

    PWM_deviation_x = -skalowanie(0,0.3,0,PWM_bias,PWM,0);
    PWM_deviation_y = -skalowanie(0,0.3,0,PWM_bias,PWM,0);
    PWM_deviation_z = skalowanie(0,0.3,0,PWM_bias,PWM,0);
    buff(i,1)=tmp(1) + rand1 + PWM_deviation_x;
    buff(i,2)=tmp(2) + rand2 + PWM_deviation_y;
    buff(i,3)=tmp(3) + rand3 + PWM_deviation_z;

    zoh=double(0);
    if(i+1>ile_probek_delay)
        mx=buff(1,1);
        my=-buff(1,2);
        mz=-buff(1,3);

    else
        mx=buff(i+1,1);
        my=-buff(i+1,2);
        mz=-buff(i+1,3);
    end

end
zoh=zoh+1;

% zamiana na gaussy tak aby moduł miał około 0.45
mod=sqrt(mx^2+my^2+mz^2);
if(mod ~= 0)
    mx_out=mx/mod*0.45;
    my_out=my/mod*0.45;
    mz_out=mz/mod*0.45;

else
    NewData = uint8(0);
    mx_out=double(0);
    my_out=double(0);
    mz_out=double(0);
end
